simulink model "USBamp_online"  (R2015a)
settings: Solver=ode45  StartTime=0.0  StopTime=Inf  RelTol=1e-3
undefined symbols (not defined in the file or in its folder): currentCFG_USBamp_online_UB, UB
libraries: dspbuff3 x2, Tools x1, gtecHighspeedLib x1, gUSBamplib x1
settings Model: Creator=Co  LastModifiedBy=Co
settings OptimizationCC: BlockReduction=off

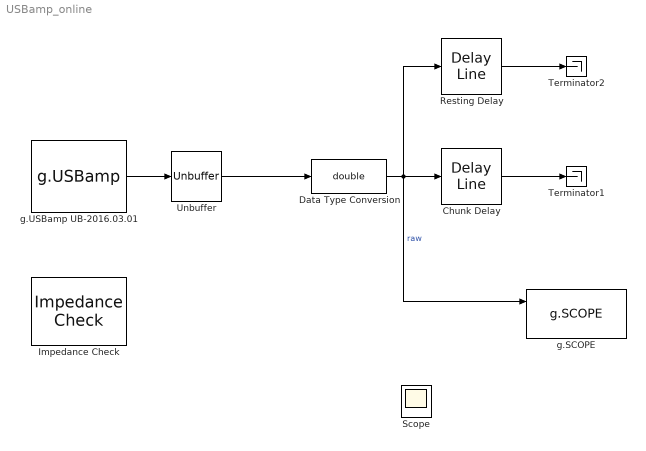
== system USBamp_online ==
  Chunk Delay : dspbuff3/Delay Line  siz=1024  ic=0  directfeed=off  enable_output=off  hold_output=off  TreatMby1Signals=M channels (this choice will be removed - see release notes)
  Data Type Conversion : DataTypeConversion  OutDataTypeStr=double
  Impedance Check : Tools/Impedance Check
  Resting Delay : dspbuff3/Delay Line  siz=512  ic=0  directfeed=off  enable_output=off  hold_output=off  TreatMby1Signals=M channels (this choice will be removed - see release notes)
  Scope : Scope
  Terminator1 : Terminator
  Terminator2 : Terminator
  Unbuffer : Unbuffer  SampleBasedProcessing=Same as frame based
  g.SCOPE : gtecHighspeedLib/g.SCOPE
  g.USBamp UB-2016.03.01 : gUSBamplib/g.USBamp  cfg=currentCFG_USBamp_online_UB-2016.03.01.cfg  snr=UB-2016.03.01
  wires:
  g.USBamp UB-2016.03.01/1 -> Unbuffer/1
  Unbuffer/1 -> Data Type Conversion/1
  Data Type Conversion/1 -> Resting Delay/1, g.SCOPE/1, Chunk Delay/1  "raw"
  Chunk Delay/1 -> Terminator1/1
  Resting Delay/1 -> Terminator2/1
